simulink subsystem "EngineDynamic"  (R2025a)
settings: Solver=VariableStepAuto  StartTime=0.0  StopTime=10.0  RelTol=1e-3
settings Model: DataDictionary=Rotor.sldd  EnableAccessToBaseWorkspace=off  Creator=LAPTOP  LastModifiedBy=LAPTOP

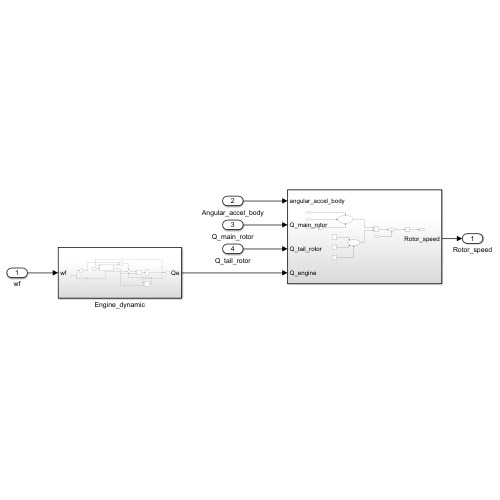
[thumbnail: Simulink's stored preview of the top-level diagram]
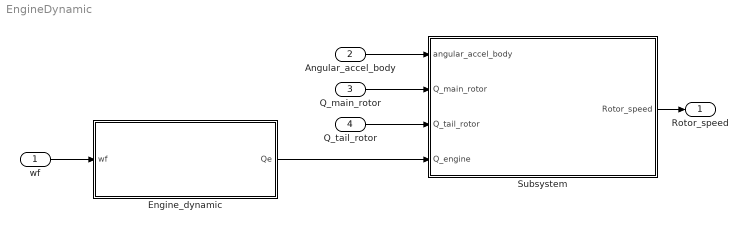
== system EngineDynamic ==
  wf : Inport
  Angular_accel_body : Inport  Port=2
  Q_main_rotor : Inport  Port=3
  Q_tail_rotor : Inport  Port=4
  Engine_dynamic : Subsystem
  Subsystem : Subsystem
  Rotor_speed : Outport
  wires:
  Engine_dynamic/1(Qe) -> Subsystem/4(Q_engine)
  wf/1 -> Engine_dynamic/1(wf)
  Subsystem/1(Rotor_speed) -> Rotor_speed/1
  Angular_accel_body/1 -> Subsystem/1(angular_accel_body)
  Q_main_rotor/1 -> Subsystem/2(Q_main_rotor)
  Q_tail_rotor/1 -> Subsystem/3(Q_tail_rotor)

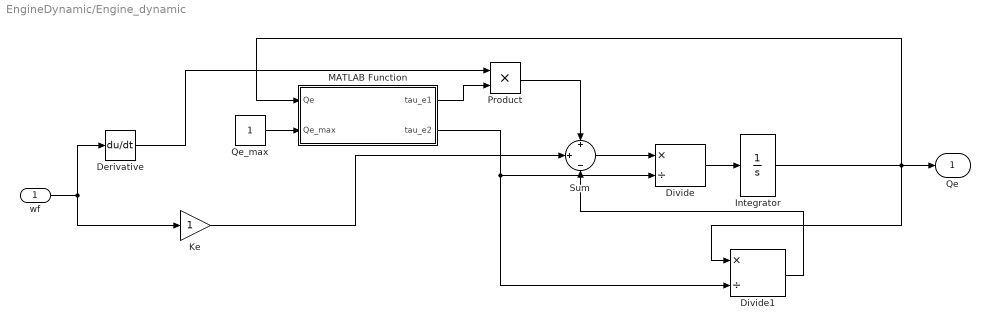
== system EngineDynamic/Engine_dynamic ==
  wf : Inport
  Derivative : Derivative
  Divide : Product  Inputs=*/
  Divide1 : Product  Inputs=*/
  Integrator : Integrator
  Ke : Gain
  MATLAB Function : MATLAB Function  TreatAsAtomicUnit=on
  Product : Product
  Qe_max : Constant
  Sum : Sum  Inputs=+|+|-
  Qe : Outport
  wires:
  wf/1 -> Ke/1, Derivative/1
  Qe_max/1 -> MATLAB Function/2(Qe_max)
  MATLAB Function/1(tau_e1) -> Product/2
  Derivative/1 -> Product/1
  Ke/1 -> Sum/2
  Product/1 -> Sum/1
  Sum/1 -> Divide/1
  MATLAB Function/2(tau_e2) -> Divide1/2, Divide/2
  Divide/1 -> Integrator/1
  Integrator/1 -> Divide1/1, Qe/1, MATLAB Function/1(Qe)
  Divide1/1 -> Sum/3

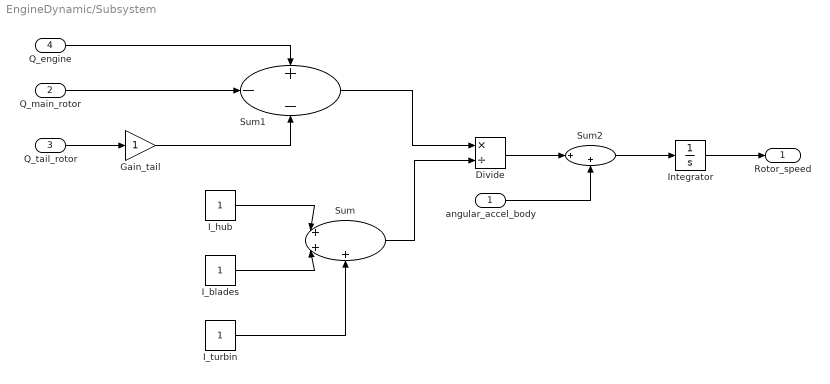
== system EngineDynamic/Subsystem ==
  angular_accel_body : Inport
  Q_main_rotor : Inport  Port=2
  Q_tail_rotor : Inport  Port=3
  Q_engine : Inport  Port=4
  Divide : Product  Inputs=*/
  Gain_tail : Gain
  I_blades : Constant
  I_hub : Constant
  I_turbin : Constant
  Integrator : Integrator
  Sum : Sum  Inputs=|+++
  Sum1 : Sum  Inputs=+--
  Sum2 : Sum  Inputs=|++
  Rotor_speed : Outport
  wires:
  Q_tail_rotor/1 -> Gain_tail/1
  I_hub/1 -> Sum/1
  I_blades/1 -> Sum/2
  I_turbin/1 -> Sum/3
  Q_engine/1 -> Sum1/1
  Q_main_rotor/1 -> Sum1/2
  Gain_tail/1 -> Sum1/3
  Sum1/1 -> Divide/1
  Sum/1 -> Divide/2
  Divide/1 -> Sum2/1
  angular_accel_body/1 -> Sum2/2
  Sum2/1 -> Integrator/1
  Integrator/1 -> Rotor_speed/1

== matlab function EngineDynamic/Engine_dynamic/MATLAB Function ==
  data: Qe input; tau_e1 output; Qe_max input; tau_e2 output
function [tau_e1, tau_e2] = calc_tau(Qe, Qe_max)
    % Qe_bar là tỷ lệ % so với Qe_max
    Qe_bar = Qe / Qe_max;
    
    tau_e1 = 0.1 - 0.03 * Qe_bar;
    tau_e2 = 0.6 - 0.5 * Qe_bar;
end
